simulink model "exampleStorage_type5"  (Simulink 8.2)
settings: Solver=ode45  StartTime=0.0  StopTime=3*3600-2  RelTol=1e-3
libraries: carnot x17, simulink x5
settings Model: Creator=drhf  LastModifiedBy=drhf
settings DataIOCC: SignalLoggingSaveFormat=Dataset
settings DebuggingCC: FcnCallInpInsideContextMsg=EnableAllAsError

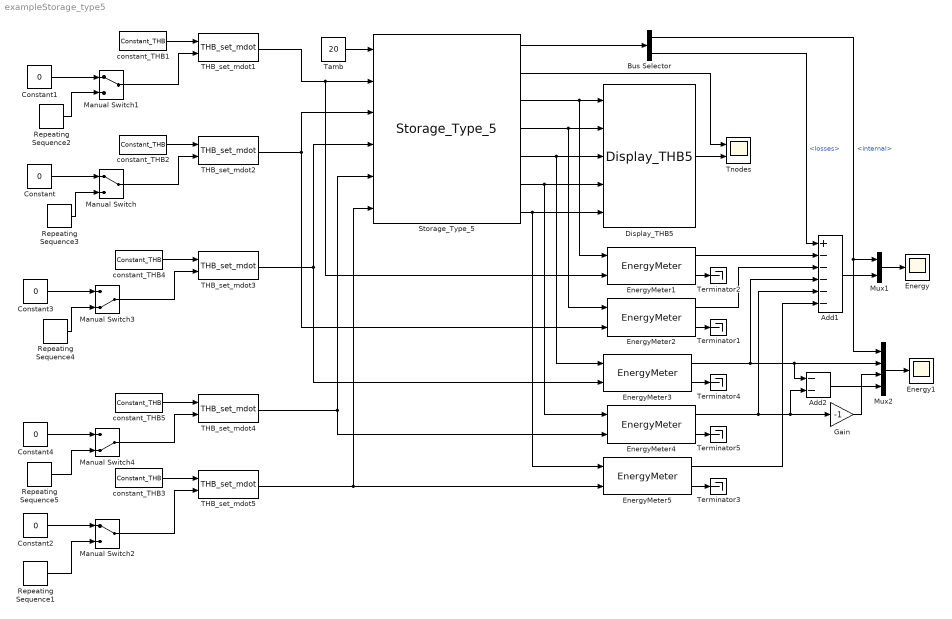
== system exampleStorage_type5 ==
  Add1 : Sum  Inputs=+-----
  Add2 : Sum  Inputs=--
  Bus Selector : BusSelector  OutputSignals=energy.internal,energy.losses
  Constant{,1..4} (5 alike) : Constant  Value=0
  Display_THB5 : carnot/Outputs/Display_THB5  t=off  m=on  p=off  id=off  mix=off  d=off
  Energy : Scope
  Energy1 : Scope
  EnergyMeter{1..5} (5 alike) : carnot/Control/EnergyMeter
  Gain : Gain  Gain=-1
  Manual Switch : ManualSwitch
  Manual Switch1 : ManualSwitch
  Manual Switch2 : ManualSwitch
  Manual Switch3 : ManualSwitch  CurrentSetting=0
  Manual Switch4 : ManualSwitch  CurrentSetting=0
  Mux1 : Mux  Inputs=2
  Mux2 : Mux
  Repeating Sequence1 : simulink/Sources/Repeating Sequence  rep_seq_t=[ 0 3600 3600+eps(3600) 7200 7200+eps(7200) 10800]  rep_seq_y=[ 0.12 0.12 0.11+0*eps(3600) 0.11 0.05+0*eps(7200) 0.05]
  Repeating Sequence2 : simulink/Sources/Repeating Sequence  rep_seq_t=[ 0 3600 3600+eps(3600) 7200 7200+eps(7200) 10440 10440+eps(10440) 11160]  rep_seq_y=[ 0 0 0.05+0*eps(3600) 0.05 0.2+0*eps(7200) 0.2 0+0*eps(10440) 0]
  Repeating Sequence3 : simulink/Sources/Repeating Sequence  rep_seq_t=[ 0 3600 3600+eps(3600) 7200 7200+eps(7200) 10800]  rep_seq_y=[ 0 0 0.1+0*eps(3600) 0.1 0.15+0*eps(7200) 0.15]
  Repeating Sequence4 : simulink/Sources/Repeating Sequence  rep_seq_t=[ 0 3600 3600+eps(3600) 7200 7200+eps(7200) 10800]  rep_seq_y=[ 0.11 0.11 0.1+0*eps(3600) 0.1 0.11+0*eps(7200) 0.11]
  Repeating Sequence5 : simulink/Sources/Repeating Sequence  rep_seq_t=[ 0 3600 3600+eps(3600) 7200 7200+eps(7200) 10800]  rep_seq_y=[ 0.12 0.12 0+0*eps(3600) 0 0.05+0*eps(7200) 0.05]
  Storage_Type_5 : carnot/Storage/Thermal/Storage_Type_5  uloss=0.74  ubot=1.37  utop=0.74  cond=0.62  t0=[10:5:55]  volume=0.75  dia=0.79  pos=standing cylinder  nconnect=5  nodes=50  mpoints=50
  THB_set_mdot{1..5} (5 alike) : carnot/Source/Simple/THB_set_mdot
  Tamb : Constant  Value=20
  Terminator{1..5} (5 alike) : Terminator
  Tnodes : Scope  NumInputPorts=2
      settings: YMin=-5~-5  YMax=5~5  SaveName=ScopeData3
  constant_THB1 : carnot/Source/Simple/Constant_THB  t=15  mdot=0*100/3600  p=1e5  mID=Full Pressure Drop with Static Height  fluid=Water  mix=0  dia=0.02  hgt=0
  constant_THB2 : carnot/Source/Simple/Constant_THB  t=60  mdot=100/3600  p=1e5  mID=Full Pressure Drop with Static Height  fluid=Water  mix=0  dia=0.02  hgt=0
  constant_THB3 : carnot/Source/Simple/Constant_THB  t=40  mdot=100/3600  p=1e5  mID=Full Pressure Drop with Static Height  fluid=Water  mix=0  dia=0.02  hgt=0
  constant_THB4 : carnot/Source/Simple/Constant_THB  t=30  mdot=100/3600  p=1e5  mID=Full Pressure Drop with Static Height  fluid=Water  mix=0  dia=0.02  hgt=0
  constant_THB5 : carnot/Source/Simple/Constant_THB  t=40  mdot=100/3600  p=1e5  mID=Full Pressure Drop with Static Height  fluid=Water  mix=0  dia=0.02  hgt=0
  wires:
  Bus Selector/1 -> Mux1/1, Mux2/1  "<internal>"
  Tamb/1 -> Storage_Type_5/1
  THB_set_mdot1/1 -> Storage_Type_5/2, EnergyMeter1/2
  THB_set_mdot2/1 -> Storage_Type_5/3, EnergyMeter2/2
  Storage_Type_5/1 -> Bus Selector/1
  Storage_Type_5/3 -> EnergyMeter1/1, Display_THB5/1
  Storage_Type_5/4 -> EnergyMeter2/1, Display_THB5/2
  Display_THB5/1 -> Tnodes/2
  Mux1/1 -> Energy/1
  EnergyMeter2/2 -> Terminator1/1
  constant_THB1/1 -> THB_set_mdot1/1
  constant_THB2/1 -> THB_set_mdot2/1
  Manual Switch1/1 -> THB_set_mdot1/2
  Manual Switch/1 -> THB_set_mdot2/2
  Constant/1 -> Manual Switch/1
  Repeating Sequence3/1 -> Manual Switch/2
  Constant1/1 -> Manual Switch1/1
  Repeating Sequence2/1 -> Manual Switch1/2
  EnergyMeter1/2 -> Terminator2/1
  Add1/1 -> Mux1/2
  EnergyMeter2/1 -> Add1/3
  EnergyMeter1/1 -> Add1/2
  constant_THB3/1 -> THB_set_mdot5/1
  Manual Switch2/1 -> THB_set_mdot5/2
  Constant2/1 -> Manual Switch2/1
  Repeating Sequence1/1 -> Manual Switch2/2
  THB_set_mdot5/1 -> Storage_Type_5/6, EnergyMeter5/2
  Storage_Type_5/2 -> Tnodes/1
  EnergyMeter5/2 -> Terminator3/1
  Storage_Type_5/5 -> EnergyMeter3/1, Display_THB5/3
  constant_THB4/1 -> THB_set_mdot3/1
  Manual Switch3/1 -> THB_set_mdot3/2
  Constant3/1 -> Manual Switch3/1
  Repeating Sequence4/1 -> Manual Switch3/2
  THB_set_mdot3/1 -> Storage_Type_5/4, EnergyMeter3/2
  EnergyMeter3/2 -> Terminator4/1
  Storage_Type_5/7 -> EnergyMeter5/1, Display_THB5/5
  constant_THB5/1 -> THB_set_mdot4/1
  Manual Switch4/1 -> THB_set_mdot4/2
  Constant4/1 -> Manual Switch4/1
  Repeating Sequence5/1 -> Manual Switch4/2
  THB_set_mdot4/1 -> Storage_Type_5/5, EnergyMeter4/2
  Storage_Type_5/6 -> EnergyMeter4/1, Display_THB5/4
  EnergyMeter5/1 -> Add1/6
  Bus Selector/2 -> Add1/1  "<losses>"
  EnergyMeter3/1 -> Add1/4, Mux2/2, Add2/1
  EnergyMeter4/2 -> Terminator5/1
  EnergyMeter4/1 -> Add1/5, Gain/1, Add2/2
  Mux2/1 -> Energy1/1
  Gain/1 -> Mux2/3
  Add2/1 -> Mux2/4
